simulink model "eg1_2011"  (Simulink 6.5)
settings: Solver=ode45  StartTime=0.0  StopTime=10.0  RelTol=1e-3
values from neighbouring files (symbols this model uses):
  B = 1    [eg1_2011_init.m]    (also in hw1p3.m = [2/R + 1/(1/(C*s)+R),-V/R,-1/(C*s+R);-1/R,0,-1/(L*s);-1/(R+1; hw1p5.m = [0, -f*s, 0; F, m*s^2+3*f*s+k, -k-f*s; 0, -f*s+k, 2*f*s+k]; hw2p1.m = [L*s+1/(C1*s), V, -L*s; -1/(C1*s), 0, 1/(C2*s); -L*s, 0, R-1; lab1.m = [1/L; 0])
  K = 1    [eg1_2011_init.m]    (also in hw7.m = 190)
  M1 = 4    [eg1_2011_init.m]
  M2 = 2    [eg1_2011_init.m]
settings Model: Creator=mct6  LastModifiedBy=mct6  ExtModeAutoUpdateStatusClock=off
settings DataIOCC: LimitDataPoints=off  SaveOutput=off  SaveTime=off  SignalLoggingName=sigsOut
settings OptimizationCC: BlockReduction=off  BooleanDataType=off
settings DebuggingCC: SolverPrmCheckMsg=none  MultiTaskDSMMsg=warning  MultiTaskCondExecSysMsg=none  StrictBusMsg=None
settings HardwareCC: TargetUnknown=on
settings RTWCC: IncludeERTFirstTime=on
settings STFCustomTargetCC: TargetFcnLib=ansi_tfl_tmw.mat  GenFloatMathFcnCalls=ANSI_C  ModelReferenceCompliant=off  SystemTargetFile=grt.tlc

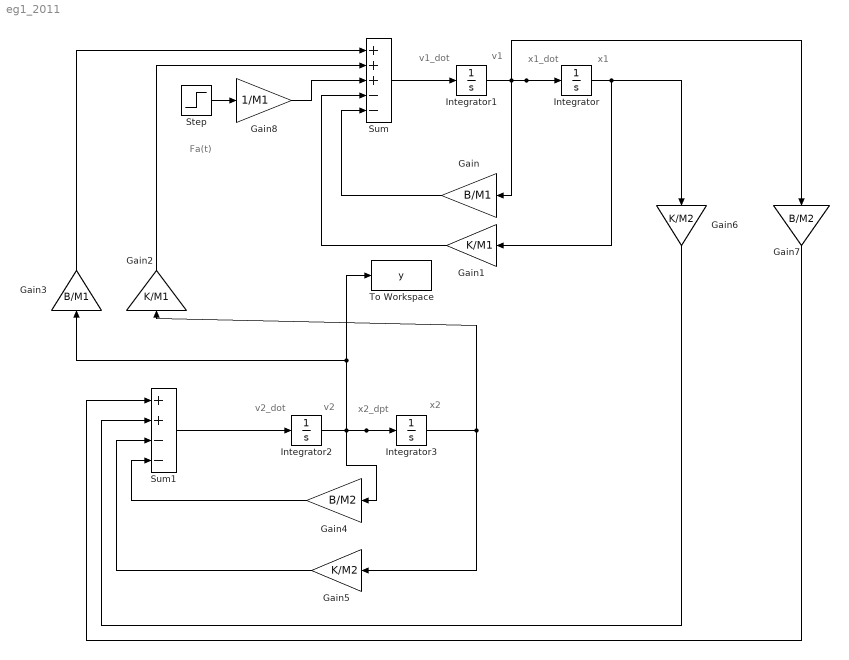
== system eg1_2011 ==
  note: Fa(t)
  note: v1_dot
  note: v1
  note: x1_dot
  note: x1
  note: v2_dot
  note: v2
  note: x2_dpt
  note: x2
  Gain : Gain  Orientation=left  Gain=B/M1  SaturateOnIntegerOverflow=on
  Gain1 : Gain  Orientation=left  Gain=K/M1  SaturateOnIntegerOverflow=on
  Gain2 : Gain  Orientation=up  Gain=K/M1  SaturateOnIntegerOverflow=on
  Gain3 : Gain  Orientation=up  Gain=B/M1  SaturateOnIntegerOverflow=on
  Gain4 : Gain  Orientation=left  Gain=B/M2  SaturateOnIntegerOverflow=on
  Gain5 : Gain  Orientation=left  Gain=K/M2  SaturateOnIntegerOverflow=on
  Gain6 : Gain  Orientation=down  Gain=K/M2  SaturateOnIntegerOverflow=on
  Gain7 : Gain  Orientation=down  Gain=B/M2  SaturateOnIntegerOverflow=on
  Gain8 : Gain  Gain=1/M1  SaturateOnIntegerOverflow=on
  Integrator{,1..3} (4 alike) : Integrator
  Step : Step  SampleTime=0
  Sum : Sum  Inputs=+++--  SaturateOnIntegerOverflow=on  InputSameDT=on
  Sum1 : Sum  Inputs=++--  SaturateOnIntegerOverflow=on  InputSameDT=on
  To Workspace : ToWorkspace  VariableName=y  SampleTime=-1  SaveFormat=Structure With Time
  wires:
  Gain6/1 -> Sum1/2
  Gain7/1 -> Sum1/1
  Sum1/1 -> Integrator2/1
  Integrator3/1 -> Gain5/1, Gain2/1
  Gain5/1 -> Sum1/3
  Gain4/1 -> Sum1/4
  Sum/1 -> Integrator1/1
  Gain1/1 -> Sum/4
  Gain/1 -> Sum/5
  Gain2/1 -> Sum/2
  Gain3/1 -> Sum/1
  Integrator2/1 -> Integrator3/1, Gain4/1, Gain3/1, To Workspace/1
  Integrator1/1 -> Gain/1, Integrator/1, Gain7/1
  Integrator/1 -> Gain1/1, Gain6/1
  Gain8/1 -> Sum/3
  Step/1 -> Gain8/1
